simulink model "EJERCICIO_b"  (Simulink 5.0)
settings: Solver=ode45  StartTime=0.0  StopTime=100  RelTol=1e-3
undefined symbols (not defined in the file): Gama
settings Model: LastModifiedBy=Administrador

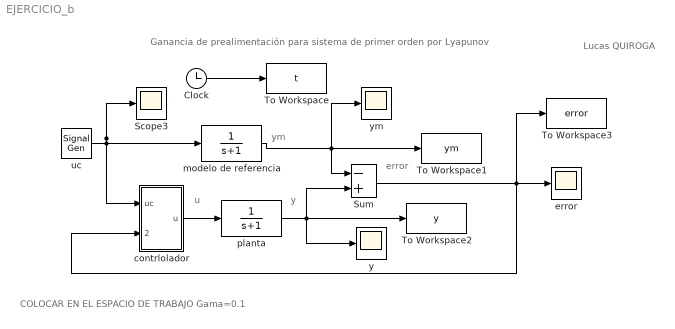
== system EJERCICIO_b ==
  note: ym
  note: y
  note: error
  note: u
  note: Ganancia de prealimentación para sistema de primer orden por Lyapunov
  note: Lucas QUIROGA
  note: COLOCAR EN EL ESPACIO DE TRABAJO
      | Gama=0.1
  Clock : Clock
  Scope3 : Scope
      settings: SaveName=ScopeData5
  Sum : Sum  Inputs=-+  SaturateOnIntegerOverflow=on
  To Workspace : ToWorkspace  VariableName=t  SampleTime=-1  SaveFormat=Array
  To Workspace1 : ToWorkspace  VariableName=ym  SampleTime=-1  SaveFormat=Array
  To Workspace2 : ToWorkspace  VariableName=y  SampleTime=-1  SaveFormat=Array
  To Workspace3 : ToWorkspace  VariableName=error  SampleTime=-1  SaveFormat=Array
  contrlolador : Subsystem
  error : Scope
      settings: SaveName=ScopeData2
  modelo de referencia : TransferFcn  Denominator=[1 1]
  planta : TransferFcn  Denominator=[1 1]
  uc : SignalGenerator  WaveForm=square  Amplitude=-1  Frequency=0.05
  y : Scope
      settings: SaveName=ScopeData4
  ym : Scope
      settings: SaveName=ScopeData3
  wires:
  Clock/1 -> To Workspace/1
  uc/1 -> contrlolador/1(uc), modelo de referencia/1, Scope3/1
  contrlolador/1(u) -> planta/1
  modelo de referencia/1 -> Sum/1, ym/1, To Workspace1/1
  planta/1 -> Sum/2, y/1, To Workspace2/1
  Sum/1 -> contrlolador/2(error), error/1, To Workspace3/1

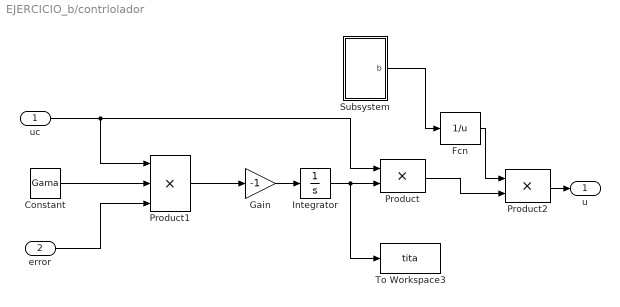
== system EJERCICIO_b/contrlolador ==
  uc : Inport
  error : Inport  Port=2
  Constant : Constant  Value=Gama
  Fcn : Fcn  Expr=1/u
  Gain : Gain  Gain=-1  SaturateOnIntegerOverflow=on
  Integrator : Integrator
  Product : Product  SaturateOnIntegerOverflow=on
  Product1 : Product  Inputs=3  SaturateOnIntegerOverflow=on
  Product2 : Product  SaturateOnIntegerOverflow=on
  Subsystem : Subsystem
  To Workspace3 : ToWorkspace  VariableName=tita  SampleTime=-1  SaveFormat=Array
  u : Outport
  wires:
  Product1/1 -> Gain/1
  Gain/1 -> Integrator/1
  Integrator/1 -> Product/2, To Workspace3/1
  Constant/1 -> Product1/2
  error/1 -> Product1/3
  uc/1 -> Product1/1, Product/1
  Subsystem/1(b) -> Fcn/1
  Product2/1 -> u/1
  Product/1 -> Product2/2
  Fcn/1 -> Product2/1

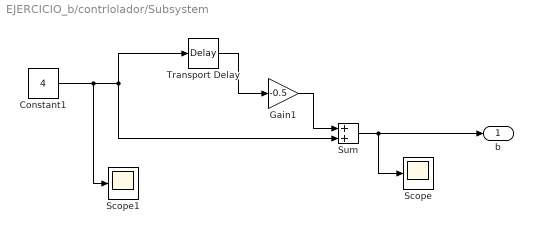
== system EJERCICIO_b/contrlolador/Subsystem ==
  Constant1 : Constant  Value=4
  Gain1 : Gain  Gain=-0.5  SaturateOnIntegerOverflow=on
  Scope : Scope
  Scope1 : Scope
  Sum : Sum  SaturateOnIntegerOverflow=on
  Transport Delay : TransportDelay  DelayTime=20
  b : Outport
  wires:
  Constant1/1 -> Sum/2, Transport Delay/1, Scope1/1
  Sum/1 -> Scope/1, b/1
  Transport Delay/1 -> Gain1/1
  Gain1/1 -> Sum/1
